simulink model "stm32_fast_serial_datalogging_host"  (R2024b)
settings: Solver=VariableStepAuto  StartTime=0.0  StopTime=100  RelTol=1e-3
libraries: instrumentseriallib x3, matrix_library x2
settings Model: PacingRate=10  Creator=The MathWorks, Inc.  LastModifiedBy=bilbe

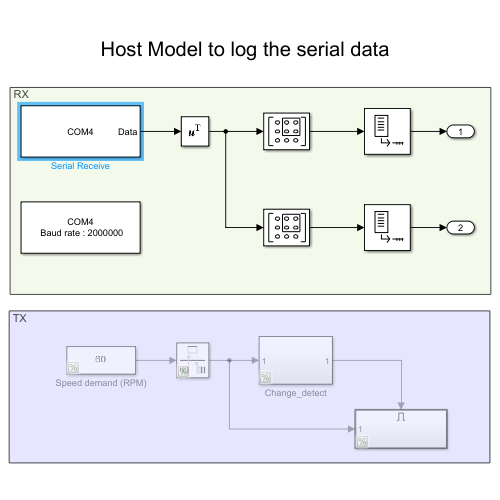
[thumbnail: Simulink's stored preview of the top-level diagram]
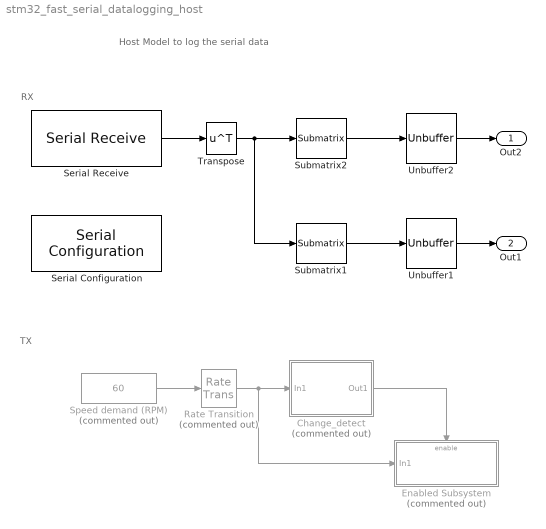
== system stm32_fast_serial_datalogging_host ==
  note: RX
  note: Host Model to log the serial data
  note: TX
  Change_detect : Subsystem  Commented=on
  Enabled Subsystem : Subsystem  Commented=on  TreatAsAtomicUnit=on
  Rate Transition : RateTransition  Commented=on  OutPortSampleTime=0.2
  Serial Configuration : instrumentseriallib/Serial Configuration  Priority=-200000  PortSel=COM4  Port=COM4  ComPort=COM4  BaudRate=2000000  DataBits=8  Parity=none  StopBits=1  ByteOrder=little-endian  FlowControl=none  Timeout=1  SimulateUsing=Interpreted execution  BlockInModel=on  aMode=1
  Serial Receive : instrumentseriallib/Serial Receive  Priority=1  PortSel=COM4  Port=COM4  ComPort=COM4  DataType=uint16  SaveDataType=uint8  ToggleHeader=on  Header=uint8('SS')  ToggleDataSize=on  DataSize=[2 600]  ToggleTerminator=on  Terminator=Custom terminator  CustomTerminator=uint8('ee')  InputFormat=Column major  EnableBlockingMode=on  ActionDataUnavailable=Output custom value  ActionWhenDataUnavailable=Output custom value  CustomValue=255  SampleTime=0.03  SimulateUsing=Interpreted execution  BlockInModel=on  aMode=1
  Speed demand (RPM) : Constant  Commented=on  Value=60  VectorParams1D=off  OutDataTypeStr=single  SampleTime=0.2
  Submatrix1 : matrix_library/Submatrix  RowSpan=All rows  RowStartMode=First  RowStartIndex=1  RowEndMode=Last  RowEndIndex=1  ColSpan=One column  ColStartMode=Last  ColStartIndex=1  ColEndMode=Last  ColEndIndex=1
  Submatrix2 : matrix_library/Submatrix  RowSpan=All rows  RowStartMode=First  RowStartIndex=1  RowEndMode=Last  RowEndIndex=1  ColSpan=One column  ColStartMode=First  ColStartIndex=1  ColEndMode=Last  ColEndIndex=1
  Transpose : Math  Operator=transpose
  Unbuffer1 : Unbuffer
  Unbuffer2 : Unbuffer
  Out2 : Outport
  Out1 : Outport  Port=2
  wires:
  Submatrix2/1 -> Unbuffer2/1
  Serial Receive/1 -> Transpose/1
  Rate Transition/1 -> Enabled Subsystem/1(In1), Change_detect/1(In1)
  Change_detect/1(Out1) -> Enabled Subsystem/Enable
  Speed demand (RPM)/1 -> Rate Transition/1
  Unbuffer1/1 -> Out1/1
  Transpose/1 -> Submatrix1/1, Submatrix2/1
  Submatrix1/1 -> Unbuffer1/1
  Unbuffer2/1 -> Out2/1

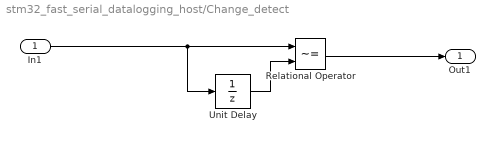
== system stm32_fast_serial_datalogging_host/Change_detect ==
  In1 : Inport
  Relational Operator : RelationalOperator  Operator=~=  OutDataTypeStr=boolean  InputSameDT=off
  Unit Delay : UnitDelay  InitialCondition=0.5  SampleTime=-1  HasFrameUpgradeWarning=on
  Out1 : Outport  VectorParamsAs1DForOutWhenUnconnected=off
  wires:
  Unit Delay/1 -> Relational Operator/2
  In1/1 -> Relational Operator/1, Unit Delay/1
  Relational Operator/1 -> Out1/1

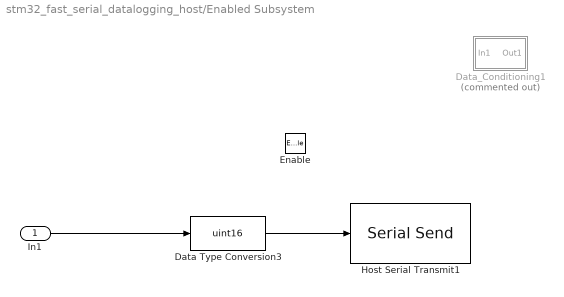
== system stm32_fast_serial_datalogging_host/Enabled Subsystem ==
  In1 : Inport
  Enable : EnablePort
  Data Type Conversion3 : DataTypeConversion  OutDataTypeStr=uint16  ConvertRealWorld=Stored Integer (SI)  RndMeth=Simplest  SaturateOnIntegerOverflow=off
  Data_Conditioning1 : Subsystem  Commented=on
  Host Serial Transmit1 : instrumentseriallib/Serial Send  PortSel=COM4  Port=COM4  ComPort=COM4  Header=[]  Terminator=<none>  CustomTerminator='E'  EnableBlockingMode=off  SimulateUsing=Interpreted execution  BlockInModel=on  aMode=5
      settings: LibrarySourceBlock=mcblib/Protection and Diagnostics/Host Serial Transmit
  wires:
  Data Type Conversion3/1 -> Host Serial Transmit1/1
  In1/1 -> Data Type Conversion3/1

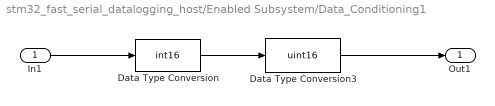
== system stm32_fast_serial_datalogging_host/Enabled Subsystem/Data_Conditioning1 ==
  In1 : Inport
  Data Type Conversion : DataTypeConversion  OutDataTypeStr=int16  RndMeth=Simplest  SaturateOnIntegerOverflow=off
  Data Type Conversion3 : DataTypeConversion  OutDataTypeStr=uint16  ConvertRealWorld=Stored Integer (SI)  RndMeth=Simplest  SaturateOnIntegerOverflow=off
  Out1 : Outport  VectorParamsAs1DForOutWhenUnconnected=off
  wires:
  Data Type Conversion/1 -> Data Type Conversion3/1
  Data Type Conversion3/1 -> Out1/1
  In1/1 -> Data Type Conversion/1
